simulink model "Simulador"  (R2015a)
settings: Solver=ode45  StartTime=0.0  StopTime=Inf  MaxStep=1  RelTol=1e-3
StopFcn:
  | close all
  | post_simulacion
model workspace (MAT data in the model file):
  m = 3.797
  b = 2.1
  c = 0.3571
  Salar = 0.75
  AR = 5.88
  cg = [0.44 0 0]
  Ix = 1.229
  Iy = 0.1702
  Iz = 0.8808
  Ixz = 0.9343
  e = 0.9935
  alpha0 = 0.267
  coefprop = [0.016415 -0.0142726]
  C_L0 = 0.0254
  C_Lalpha = 4.0191
  C_Lq = 3.8954
  C_Ldelta_e = 0.5872
  C_D0 = 0.0102
  C_Dbeta1 = -2.0864e-07
  C_Dbeta2 = 0.0671
  C_Dq = 0
  C_Ddelta_e = 0.8461
  C_Y0 = 3.2049e-18
  C_Ybeta = -0.1949
  C_Yp = -0.1172
  C_Yr = 0.0959
  C_Ydelta_a = -0.0696
  C_l0 = 1.1518e-18
  C_lbeta = -0.0765
  C_lp = -0.4018
  C_lr = 0.025
  C_ldelta_a = 0.2987
  C_m0 = 0.018
  C_malpha = -0.2524
  C_mq = -1.3047
  C_mdelta_e = -0.4857
  C_n0 = -2.2667e-07
  C_nbeta = 0.0403
  C_np = -0.0247
  C_nr = -0.1252
  C_ndelta_a = 0.0076
  gamma = 0.20958671
  gamma1 = 8.64638926772
  gamma2 = 7.15127867602
  gamma3 = 4.20255654569
  gamma4 = 4.4578208227
  gamma5 = -2.04582843713
  gamma6 = 5.48942420682
  gamma7 = 10.3736620037
  gamma8 = 5.86392142899
  C_p0 = -1.01045424588e-06
  C_pbeta = -0.14184539659
  C_pp = -1.79869539438
  C_pr = -0.45305525336
  C_pdelta_a = 1.28918307845
  C_r0 = -1.3291750703e-06
  C_rbeta = -0.104707259349
  C_rp = -1.93599126586
  C_rr = -0.622717442342
  C_rdelta_a = 1.3761168826
  C_mp = -0.2168
values from neighbouring files (symbols this model uses):
  r = [r_n;r_e;r_d]    [segmento.m]
  waypoints = reshape(waypoints_mat.',[],1)    [plan_de_vuelo.m]
undefined symbols (not defined in the file or in its folder): F, Light, magnitude, MIL, plan_de_vuelo
libraries: simulink_extras x20, aerolibconvert2 x18, aerolibfltsims x2, simulink x2, vrlib x1, instrumentlib x1, aerolibatmos2 x1, aerolibtransform2 x1, aerolibwind2 x1, aerolibgravity2 x1
(part 3 of 3)

== system Simulador/Autopiloto/Activador de controladores/Interruptor con latch/Memoria de pulsacion del teclado ==
  Estado del boton : Inport
  Reinicio : Inport  Port=2
  Activador : EnablePort
  Interruptor : Switch  Threshold=1
  Latch D : simulink_extras/Flip Flops/D Latch
  Memoria : Memory
  Operador logico : Logic  Operator=XOR  AllPortsSameDT=off  OutDataTypeStr=boolean
  Operador logico1 : Logic  AllPortsSameDT=off  OutDataTypeStr=boolean
  Operador logico2 : Logic  Operator=NOT  AllPortsSameDT=off  OutDataTypeStr=boolean
  Terminador : Terminator
  Tierra : Ground
  Estado del controlador : Outport
  wires:
  Operador logico2/1 -> Latch D/1
  Memoria/1 -> Operador logico2/1, Operador logico1/2
  Tierra/1 -> Interruptor/3
  Latch D/2 -> Terminador/1
  Estado del boton/1 -> Interruptor/2, Interruptor/1
  Latch D/1 -> Estado del controlador/1, Memoria/1
  Operador logico/1 -> Latch D/2
  Interruptor/1 -> Operador logico/1
  Reinicio/1 -> Operador logico1/1
  Operador logico1/1 -> Operador logico/2

== system Simulador/Autopiloto/Activador de controladores/Interruptor con latch1/Memoria de pulsacion del joystick ==
  Estado del boton : Inport
  Reinicio : Inport  Port=2
  Activador : EnablePort
  Interruptor1 : Switch  Criteria=u2 > Threshold
  Interruptor2 : Switch  Criteria=u2 > Threshold
  Latch D : simulink_extras/Flip Flops/D Latch
  Operador logico : Logic  Operator=NOT  AllPortsSameDT=off  OutDataTypeStr=boolean
  Operador logico1 : Logic  Operator=NOT  AllPortsSameDT=off  OutDataTypeStr=boolean
  Operador logico2 : Logic  Operator=XOR  AllPortsSameDT=off  OutDataTypeStr=boolean
  Retraso : Delay  DelayLength=1  InitialCondition=0  SampleTime=0.5
  Terminador : Terminator
  Estado del controlador : Outport
  wires:
  Latch D/2 -> Terminador/1
  Latch D/1 -> Retraso/1, Estado del controlador/1
  Operador logico/1 -> Interruptor1/1
  Retraso/1 -> Interruptor1/2
  Estado del boton/1 -> Operador logico/1, Interruptor1/3, Operador logico2/1
  Interruptor2/1 -> Latch D/1
  Interruptor1/1 -> Interruptor2/3
  Operador logico1/1 -> Interruptor2/1
  Operador logico2/1 -> Latch D/2
  Reinicio/1 -> Interruptor2/2, Operador logico1/1, Operador logico2/2

== system Simulador/Autopiloto/Activador de controladores/Interruptor con latch1/Memoria de pulsacion del teclado ==
  Estado del boton : Inport
  Reinicio : Inport  Port=2
  Activador : EnablePort
  Interruptor : Switch  Threshold=1
  Latch D : simulink_extras/Flip Flops/D Latch
  Memoria : Memory
  Operador logico : Logic  Operator=XOR  AllPortsSameDT=off  OutDataTypeStr=boolean
  Operador logico1 : Logic  AllPortsSameDT=off  OutDataTypeStr=boolean
  Operador logico2 : Logic  Operator=NOT  AllPortsSameDT=off  OutDataTypeStr=boolean
  Terminador : Terminator
  Tierra : Ground
  Estado del controlador : Outport
  wires:
  Operador logico2/1 -> Latch D/1
  Memoria/1 -> Operador logico2/1, Operador logico1/2
  Tierra/1 -> Interruptor/3
  Latch D/2 -> Terminador/1
  Estado del boton/1 -> Interruptor/2, Interruptor/1
  Latch D/1 -> Estado del controlador/1, Memoria/1
  Operador logico/1 -> Latch D/2
  Interruptor/1 -> Operador logico/1
  Reinicio/1 -> Operador logico1/1
  Operador logico1/1 -> Operador logico/2

== system Simulador/Autopiloto/Activador de controladores/Interruptor con latch2/Memoria de pulsacion del joystick ==
  Estado del boton : Inport
  Reinicio : Inport  Port=2
  Activador : EnablePort
  Interruptor1 : Switch  Criteria=u2 > Threshold
  Interruptor2 : Switch  Criteria=u2 > Threshold
  Latch D : simulink_extras/Flip Flops/D Latch
  Operador logico : Logic  Operator=NOT  AllPortsSameDT=off  OutDataTypeStr=boolean
  Operador logico1 : Logic  Operator=NOT  AllPortsSameDT=off  OutDataTypeStr=boolean
  Operador logico2 : Logic  Operator=XOR  AllPortsSameDT=off  OutDataTypeStr=boolean
  Retraso : Delay  DelayLength=1  InitialCondition=0  SampleTime=0.5
  Terminador : Terminator
  Estado del controlador : Outport
  wires:
  Latch D/2 -> Terminador/1
  Latch D/1 -> Retraso/1, Estado del controlador/1
  Operador logico/1 -> Interruptor1/1
  Retraso/1 -> Interruptor1/2
  Estado del boton/1 -> Operador logico/1, Interruptor1/3, Operador logico2/1
  Interruptor2/1 -> Latch D/1
  Interruptor1/1 -> Interruptor2/3
  Operador logico1/1 -> Interruptor2/1
  Operador logico2/1 -> Latch D/2
  Reinicio/1 -> Interruptor2/2, Operador logico1/1, Operador logico2/2

== system Simulador/Autopiloto/Activador de controladores/Interruptor con latch2/Memoria de pulsacion del teclado ==
  Estado del boton : Inport
  Reinicio : Inport  Port=2
  Activador : EnablePort
  Interruptor : Switch  Threshold=1
  Latch D : simulink_extras/Flip Flops/D Latch
  Memoria : Memory
  Operador logico : Logic  Operator=XOR  AllPortsSameDT=off  OutDataTypeStr=boolean
  Operador logico1 : Logic  AllPortsSameDT=off  OutDataTypeStr=boolean
  Operador logico2 : Logic  Operator=NOT  AllPortsSameDT=off  OutDataTypeStr=boolean
  Terminador : Terminator
  Tierra : Ground
  Estado del controlador : Outport
  wires:
  Operador logico2/1 -> Latch D/1
  Memoria/1 -> Operador logico2/1, Operador logico1/2
  Tierra/1 -> Interruptor/3
  Latch D/2 -> Terminador/1
  Estado del boton/1 -> Interruptor/2, Interruptor/1
  Latch D/1 -> Estado del controlador/1, Memoria/1
  Operador logico/1 -> Latch D/2
  Interruptor/1 -> Operador logico/1
  Reinicio/1 -> Operador logico1/1
  Operador logico1/1 -> Operador logico/2

== system Simulador/Autopiloto/Activador de controladores/Interruptor con latch3/Memoria de pulsacion del joystick ==
  Estado del boton : Inport
  Reinicio : Inport  Port=2
  Activador : EnablePort
  Interruptor1 : Switch  Criteria=u2 > Threshold
  Interruptor2 : Switch  Criteria=u2 > Threshold
  Latch D : simulink_extras/Flip Flops/D Latch
  Operador logico : Logic  Operator=NOT  AllPortsSameDT=off  OutDataTypeStr=boolean
  Operador logico1 : Logic  Operator=NOT  AllPortsSameDT=off  OutDataTypeStr=boolean
  Operador logico2 : Logic  Operator=XOR  AllPortsSameDT=off  OutDataTypeStr=boolean
  Retraso : Delay  DelayLength=1  InitialCondition=0  SampleTime=0.5
  Terminador : Terminator
  Estado del controlador : Outport
  wires:
  Latch D/2 -> Terminador/1
  Latch D/1 -> Retraso/1, Estado del controlador/1
  Operador logico/1 -> Interruptor1/1
  Retraso/1 -> Interruptor1/2
  Estado del boton/1 -> Operador logico/1, Interruptor1/3, Operador logico2/1
  Interruptor2/1 -> Latch D/1
  Interruptor1/1 -> Interruptor2/3
  Operador logico1/1 -> Interruptor2/1
  Operador logico2/1 -> Latch D/2
  Reinicio/1 -> Interruptor2/2, Operador logico1/1, Operador logico2/2

== system Simulador/Autopiloto/Activador de controladores/Interruptor con latch3/Memoria de pulsacion del teclado ==
  Estado del boton : Inport
  Reinicio : Inport  Port=2
  Activador : EnablePort
  Interruptor : Switch  Threshold=1
  Latch D : simulink_extras/Flip Flops/D Latch
  Memoria : Memory
  Operador logico : Logic  Operator=XOR  AllPortsSameDT=off  OutDataTypeStr=boolean
  Operador logico1 : Logic  AllPortsSameDT=off  OutDataTypeStr=boolean
  Operador logico2 : Logic  Operator=NOT  AllPortsSameDT=off  OutDataTypeStr=boolean
  Terminador : Terminator
  Tierra : Ground
  Estado del controlador : Outport
  wires:
  Operador logico2/1 -> Latch D/1
  Memoria/1 -> Operador logico2/1, Operador logico1/2
  Tierra/1 -> Interruptor/3
  Latch D/2 -> Terminador/1
  Estado del boton/1 -> Interruptor/2, Interruptor/1
  Latch D/1 -> Estado del controlador/1, Memoria/1
  Operador logico/1 -> Latch D/2
  Interruptor/1 -> Operador logico/1
  Reinicio/1 -> Operador logico1/1
  Operador logico1/1 -> Operador logico/2

== system Simulador/Autopiloto/Activador de controladores/Interruptor con latch4/Memoria de pulsacion del joystick ==
  Estado del boton : Inport
  Reinicio : Inport  Port=2
  Activador : EnablePort
  Interruptor1 : Switch  Criteria=u2 > Threshold
  Interruptor2 : Switch  Criteria=u2 > Threshold
  Latch D : simulink_extras/Flip Flops/D Latch
  Operador logico : Logic  Operator=NOT  AllPortsSameDT=off  OutDataTypeStr=boolean
  Operador logico1 : Logic  Operator=NOT  AllPortsSameDT=off  OutDataTypeStr=boolean
  Operador logico2 : Logic  Operator=XOR  AllPortsSameDT=off  OutDataTypeStr=boolean
  Retraso : Delay  DelayLength=1  InitialCondition=0  SampleTime=0.5
  Terminador : Terminator
  Estado del controlador : Outport
  wires:
  Latch D/2 -> Terminador/1
  Latch D/1 -> Retraso/1, Estado del controlador/1
  Operador logico/1 -> Interruptor1/1
  Retraso/1 -> Interruptor1/2
  Estado del boton/1 -> Operador logico/1, Interruptor1/3, Operador logico2/1
  Interruptor2/1 -> Latch D/1
  Interruptor1/1 -> Interruptor2/3
  Operador logico1/1 -> Interruptor2/1
  Operador logico2/1 -> Latch D/2
  Reinicio/1 -> Interruptor2/2, Operador logico1/1, Operador logico2/2

== system Simulador/Autopiloto/Activador de controladores/Interruptor con latch4/Memoria de pulsacion del teclado ==
  Estado del boton : Inport
  Reinicio : Inport  Port=2
  Activador : EnablePort
  Interruptor : Switch  Threshold=1
  Latch D : simulink_extras/Flip Flops/D Latch
  Memoria : Memory
  Operador logico : Logic  Operator=XOR  AllPortsSameDT=off  OutDataTypeStr=boolean
  Operador logico1 : Logic  AllPortsSameDT=off  OutDataTypeStr=boolean
  Operador logico2 : Logic  Operator=NOT  AllPortsSameDT=off  OutDataTypeStr=boolean
  Terminador : Terminator
  Tierra : Ground
  Estado del controlador : Outport
  wires:
  Operador logico2/1 -> Latch D/1
  Memoria/1 -> Operador logico2/1, Operador logico1/2
  Tierra/1 -> Interruptor/3
  Latch D/2 -> Terminador/1
  Estado del boton/1 -> Interruptor/2, Interruptor/1
  Latch D/1 -> Estado del controlador/1, Memoria/1
  Operador logico/1 -> Latch D/2
  Interruptor/1 -> Operador logico/1
  Reinicio/1 -> Operador logico1/1
  Operador logico1/1 -> Operador logico/2

== system Simulador/Autopiloto/Activador de controladores/Interruptor con latch5/Memoria de pulsacion del joystick ==
  Estado del boton : Inport
  Reinicio : Inport  Port=2
  Activador : EnablePort
  Interruptor1 : Switch  Criteria=u2 > Threshold
  Interruptor2 : Switch  Criteria=u2 > Threshold
  Latch D : simulink_extras/Flip Flops/D Latch
  Operador logico : Logic  Operator=NOT  AllPortsSameDT=off  OutDataTypeStr=boolean
  Operador logico1 : Logic  Operator=NOT  AllPortsSameDT=off  OutDataTypeStr=boolean
  Operador logico2 : Logic  Operator=XOR  AllPortsSameDT=off  OutDataTypeStr=boolean
  Retraso : Delay  DelayLength=1  InitialCondition=0  SampleTime=0.5
  Terminador : Terminator
  Estado del controlador : Outport
  wires:
  Latch D/2 -> Terminador/1
  Latch D/1 -> Retraso/1, Estado del controlador/1
  Operador logico/1 -> Interruptor1/1
  Retraso/1 -> Interruptor1/2
  Estado del boton/1 -> Operador logico/1, Interruptor1/3, Operador logico2/1
  Interruptor2/1 -> Latch D/1
  Interruptor1/1 -> Interruptor2/3
  Operador logico1/1 -> Interruptor2/1
  Operador logico2/1 -> Latch D/2
  Reinicio/1 -> Interruptor2/2, Operador logico1/1, Operador logico2/2

== system Simulador/Autopiloto/Activador de controladores/Interruptor con latch5/Memoria de pulsacion del teclado ==
  Estado del boton : Inport
  Reinicio : Inport  Port=2
  Activador : EnablePort
  Interruptor : Switch  Threshold=1
  Latch D : simulink_extras/Flip Flops/D Latch
  Memoria : Memory
  Operador logico : Logic  Operator=XOR  AllPortsSameDT=off  OutDataTypeStr=boolean
  Operador logico1 : Logic  AllPortsSameDT=off  OutDataTypeStr=boolean
  Operador logico2 : Logic  Operator=NOT  AllPortsSameDT=off  OutDataTypeStr=boolean
  Terminador : Terminator
  Tierra : Ground
  Estado del controlador : Outport
  wires:
  Operador logico2/1 -> Latch D/1
  Memoria/1 -> Operador logico2/1, Operador logico1/2
  Tierra/1 -> Interruptor/3
  Latch D/2 -> Terminador/1
  Estado del boton/1 -> Interruptor/2, Interruptor/1
  Latch D/1 -> Estado del controlador/1, Memoria/1
  Operador logico/1 -> Latch D/2
  Interruptor/1 -> Operador logico/1
  Reinicio/1 -> Operador logico1/1
  Operador logico1/1 -> Operador logico/2

== system Simulador/Autopiloto/Activador de controladores/Interruptor con latch6/Memoria de pulsacion del joystick ==
  Estado del boton : Inport
  Reinicio : Inport  Port=2
  Activador : EnablePort
  Interruptor1 : Switch  Criteria=u2 > Threshold
  Interruptor2 : Switch  Criteria=u2 > Threshold
  Latch D : simulink_extras/Flip Flops/D Latch
  Operador logico : Logic  Operator=NOT  AllPortsSameDT=off  OutDataTypeStr=boolean
  Operador logico1 : Logic  Operator=NOT  AllPortsSameDT=off  OutDataTypeStr=boolean
  Operador logico2 : Logic  Operator=XOR  AllPortsSameDT=off  OutDataTypeStr=boolean
  Retraso : Delay  DelayLength=1  InitialCondition=0  SampleTime=0.5
  Terminador : Terminator
  Estado del controlador : Outport
  wires:
  Latch D/2 -> Terminador/1
  Latch D/1 -> Retraso/1, Estado del controlador/1
  Operador logico/1 -> Interruptor1/1
  Retraso/1 -> Interruptor1/2
  Estado del boton/1 -> Operador logico/1, Interruptor1/3, Operador logico2/1
  Interruptor2/1 -> Latch D/1
  Interruptor1/1 -> Interruptor2/3
  Operador logico1/1 -> Interruptor2/1
  Operador logico2/1 -> Latch D/2
  Reinicio/1 -> Interruptor2/2, Operador logico1/1, Operador logico2/2

== system Simulador/Autopiloto/Activador de controladores/Interruptor con latch6/Memoria de pulsacion del teclado ==
  Estado del boton : Inport
  Reinicio : Inport  Port=2
  Activador : EnablePort
  Interruptor : Switch  Threshold=1
  Latch D : simulink_extras/Flip Flops/D Latch
  Memoria : Memory
  Operador logico : Logic  Operator=XOR  AllPortsSameDT=off  OutDataTypeStr=boolean
  Operador logico1 : Logic  AllPortsSameDT=off  OutDataTypeStr=boolean
  Operador logico2 : Logic  Operator=NOT  AllPortsSameDT=off  OutDataTypeStr=boolean
  Terminador : Terminator
  Tierra : Ground
  Estado del controlador : Outport
  wires:
  Operador logico2/1 -> Latch D/1
  Memoria/1 -> Operador logico2/1, Operador logico1/2
  Tierra/1 -> Interruptor/3
  Latch D/2 -> Terminador/1
  Estado del boton/1 -> Interruptor/2, Interruptor/1
  Latch D/1 -> Estado del controlador/1, Memoria/1
  Operador logico/1 -> Latch D/2
  Interruptor/1 -> Operador logico/1
  Reinicio/1 -> Operador logico1/1
  Operador logico1/1 -> Operador logico/2

== system Simulador/Autopiloto/Activador de controladores/Interruptor con latch7/Memoria de pulsacion del joystick ==
  Estado del boton : Inport
  Reinicio : Inport  Port=2
  Activador : EnablePort
  Interruptor1 : Switch  Criteria=u2 > Threshold
  Interruptor2 : Switch  Criteria=u2 > Threshold
  Latch D : simulink_extras/Flip Flops/D Latch
  Operador logico : Logic  Operator=NOT  AllPortsSameDT=off  OutDataTypeStr=boolean
  Operador logico1 : Logic  Operator=NOT  AllPortsSameDT=off  OutDataTypeStr=boolean
  Operador logico2 : Logic  Operator=XOR  AllPortsSameDT=off  OutDataTypeStr=boolean
  Retraso : Delay  DelayLength=1  InitialCondition=0  SampleTime=0.5
  Terminador : Terminator
  Estado del controlador : Outport
  wires:
  Latch D/2 -> Terminador/1
  Latch D/1 -> Retraso/1, Estado del controlador/1
  Operador logico/1 -> Interruptor1/1
  Retraso/1 -> Interruptor1/2
  Estado del boton/1 -> Operador logico/1, Interruptor1/3, Operador logico2/1
  Interruptor2/1 -> Latch D/1
  Interruptor1/1 -> Interruptor2/3
  Operador logico1/1 -> Interruptor2/1
  Operador logico2/1 -> Latch D/2
  Reinicio/1 -> Interruptor2/2, Operador logico1/1, Operador logico2/2

== system Simulador/Autopiloto/Activador de controladores/Interruptor con latch7/Memoria de pulsacion del teclado ==
  Estado del boton : Inport
  Reinicio : Inport  Port=2
  Activador : EnablePort
  Interruptor : Switch  Threshold=1
  Latch D : simulink_extras/Flip Flops/D Latch
  Memoria : Memory
  Operador logico : Logic  Operator=XOR  AllPortsSameDT=off  OutDataTypeStr=boolean
  Operador logico1 : Logic  AllPortsSameDT=off  OutDataTypeStr=boolean
  Operador logico2 : Logic  Operator=NOT  AllPortsSameDT=off  OutDataTypeStr=boolean
  Terminador : Terminator
  Tierra : Ground
  Estado del controlador : Outport
  wires:
  Operador logico2/1 -> Latch D/1
  Memoria/1 -> Operador logico2/1, Operador logico1/2
  Tierra/1 -> Interruptor/3
  Latch D/2 -> Terminador/1
  Estado del boton/1 -> Interruptor/2, Interruptor/1
  Latch D/1 -> Estado del controlador/1, Memoria/1
  Operador logico/1 -> Latch D/2
  Interruptor/1 -> Operador logico/1
  Reinicio/1 -> Operador logico1/1
  Operador logico1/1 -> Operador logico/2

== system Simulador/Autopiloto/Activador de controladores/Interruptor con latch8/Memoria de pulsacion del joystick ==
  Estado del boton : Inport
  Reinicio : Inport  Port=2
  Activador : EnablePort
  Interruptor1 : Switch  Criteria=u2 > Threshold
  Interruptor2 : Switch  Criteria=u2 > Threshold
  Latch D : simulink_extras/Flip Flops/D Latch
  Operador logico : Logic  Operator=NOT  AllPortsSameDT=off  OutDataTypeStr=boolean
  Operador logico1 : Logic  Operator=NOT  AllPortsSameDT=off  OutDataTypeStr=boolean
  Operador logico2 : Logic  Operator=XOR  AllPortsSameDT=off  OutDataTypeStr=boolean
  Retraso : Delay  DelayLength=1  InitialCondition=0  SampleTime=0.5
  Terminador : Terminator
  Estado del controlador : Outport
  wires:
  Latch D/2 -> Terminador/1
  Latch D/1 -> Retraso/1, Estado del controlador/1
  Operador logico/1 -> Interruptor1/1
  Retraso/1 -> Interruptor1/2
  Estado del boton/1 -> Operador logico/1, Interruptor1/3, Operador logico2/1
  Interruptor2/1 -> Latch D/1
  Interruptor1/1 -> Interruptor2/3
  Operador logico1/1 -> Interruptor2/1
  Operador logico2/1 -> Latch D/2
  Reinicio/1 -> Interruptor2/2, Operador logico1/1, Operador logico2/2

== system Simulador/Autopiloto/Activador de controladores/Interruptor con latch8/Memoria de pulsacion del teclado ==
  Estado del boton : Inport
  Reinicio : Inport  Port=2
  Activador : EnablePort
  Interruptor : Switch  Threshold=1
  Latch D : simulink_extras/Flip Flops/D Latch
  Memoria : Memory
  Operador logico : Logic  Operator=XOR  AllPortsSameDT=off  OutDataTypeStr=boolean
  Operador logico1 : Logic  AllPortsSameDT=off  OutDataTypeStr=boolean
  Operador logico2 : Logic  Operator=NOT  AllPortsSameDT=off  OutDataTypeStr=boolean
  Terminador : Terminator
  Tierra : Ground
  Estado del controlador : Outport
  wires:
  Operador logico2/1 -> Latch D/1
  Memoria/1 -> Operador logico2/1, Operador logico1/2
  Tierra/1 -> Interruptor/3
  Latch D/2 -> Terminador/1
  Estado del boton/1 -> Interruptor/2, Interruptor/1
  Latch D/1 -> Estado del controlador/1, Memoria/1
  Operador logico/1 -> Latch D/2
  Interruptor/1 -> Operador logico/1
  Reinicio/1 -> Operador logico1/1
  Operador logico1/1 -> Operador logico/2

== system Simulador/Autopiloto/Activador de controladores/Interruptor con latch9/Memoria de pulsacion del joystick ==
  Estado del boton : Inport
  Reinicio : Inport  Port=2
  Activador : EnablePort
  Interruptor1 : Switch  Criteria=u2 > Threshold
  Interruptor2 : Switch  Criteria=u2 > Threshold
  Latch D : simulink_extras/Flip Flops/D Latch
  Operador logico : Logic  Operator=NOT  AllPortsSameDT=off  OutDataTypeStr=boolean
  Operador logico1 : Logic  Operator=NOT  AllPortsSameDT=off  OutDataTypeStr=boolean
  Operador logico2 : Logic  Operator=XOR  AllPortsSameDT=off  OutDataTypeStr=boolean
  Retraso : Delay  DelayLength=1  InitialCondition=0  SampleTime=0.5
  Terminador : Terminator
  Estado del controlador : Outport
  wires:
  Latch D/2 -> Terminador/1
  Latch D/1 -> Retraso/1, Estado del controlador/1
  Operador logico/1 -> Interruptor1/1
  Retraso/1 -> Interruptor1/2
  Estado del boton/1 -> Operador logico/1, Interruptor1/3, Operador logico2/1
  Interruptor2/1 -> Latch D/1
  Interruptor1/1 -> Interruptor2/3
  Operador logico1/1 -> Interruptor2/1
  Operador logico2/1 -> Latch D/2
  Reinicio/1 -> Interruptor2/2, Operador logico1/1, Operador logico2/2

== system Simulador/Autopiloto/Activador de controladores/Interruptor con latch9/Memoria de pulsacion del teclado ==
  Estado del boton : Inport
  Reinicio : Inport  Port=2
  Activador : EnablePort
  Interruptor : Switch  Threshold=1
  Latch D : simulink_extras/Flip Flops/D Latch
  Memoria : Memory
  Operador logico : Logic  Operator=XOR  AllPortsSameDT=off  OutDataTypeStr=boolean
  Operador logico1 : Logic  AllPortsSameDT=off  OutDataTypeStr=boolean
  Operador logico2 : Logic  Operator=NOT  AllPortsSameDT=off  OutDataTypeStr=boolean
  Terminador : Terminator
  Tierra : Ground
  Estado del controlador : Outport
  wires:
  Operador logico2/1 -> Latch D/1
  Memoria/1 -> Operador logico2/1, Operador logico1/2
  Tierra/1 -> Interruptor/3
  Latch D/2 -> Terminador/1
  Estado del boton/1 -> Interruptor/2, Interruptor/1
  Latch D/1 -> Estado del controlador/1, Memoria/1
  Operador logico/1 -> Latch D/2
  Interruptor/1 -> Operador logico/1
  Reinicio/1 -> Operador logico1/1
  Operador logico1/1 -> Operador logico/2

== system Simulador/Entrada de control manual/Teclado/Reconocedor de teclado/Subsistema de accion del interruptor de eventos ==
  Eje alerones : Inport
  Tecla : Inport  Port=2
  Puerto de accion : ActionPort  ActionType=case
  Constante : Constant  Value=0.05
  Constante1 : Constant  Value=-0.05
  Interruptor : Switch  Criteria=u2 > Threshold  Threshold=97
  Saturacion : Saturate  UpperLimit=1  LowerLimit=-1
  Sum : Sum  Inputs=|++
  Eje alerones_ : Outport
  wires:
  Tecla/1 -> Interruptor/2
  Constante1/1 -> Interruptor/3
  Constante/1 -> Interruptor/1
  Eje alerones/1 -> Sum/1
  Interruptor/1 -> Sum/2
  Sum/1 -> Saturacion/1
  Saturacion/1 -> Eje alerones_/1

== system Simulador/Entrada de control manual/Teclado/Reconocedor de teclado/Subsistema de accion del interruptor de eventos1 ==
  Eje elevadores : Inport
  Tecla : Inport  Port=2
  Puerto de accion : ActionPort  ActionType=case
  Constante : Constant  Value=0.05
  Constante1 : Constant  Value=-0.05
  Interruptor : Switch  Criteria=u2 > Threshold  Threshold=115
  Saturacion : Saturate  UpperLimit=1  LowerLimit=-1
  Sum : Sum  Inputs=|++
  Eje elevadores_ : Outport
  wires:
  Eje elevadores/1 -> Sum/1
  Interruptor/1 -> Sum/2
  Sum/1 -> Saturacion/1
  Saturacion/1 -> Eje elevadores_/1
  Tecla/1 -> Interruptor/2
  Constante/1 -> Interruptor/1
  Constante1/1 -> Interruptor/3

== system Simulador/Entrada de control manual/Teclado/Reconocedor de teclado/Subsistema de accion del interruptor de eventos10 ==
  Pulsacion : Inport  PortDimensions=1
  Puerto de accion : ActionPort  ActionType=case
  Boton_ : Outport
  wires:
  Pulsacion/1 -> Boton_/1

== system Simulador/Entrada de control manual/Teclado/Reconocedor de teclado/Subsistema de accion del interruptor de eventos11 ==
  Pulsacion : Inport  PortDimensions=1
  Puerto de accion : ActionPort  ActionType=case
  Boton_ : Outport
  wires:
  Pulsacion/1 -> Boton_/1

== system Simulador/Entrada de control manual/Teclado/Reconocedor de teclado/Subsistema de accion del interruptor de eventos12 ==
  Pulsacion : Inport  PortDimensions=1
  Puerto de accion : ActionPort  ActionType=case
  Boton_ : Outport
  wires:
  Pulsacion/1 -> Boton_/1

== system Simulador/Entrada de control manual/Teclado/Reconocedor de teclado/Subsistema de accion del interruptor de eventos13 ==
  Pulsacion : Inport  PortDimensions=1
  Puerto de accion : ActionPort  ActionType=case
  Boton_ : Outport
  wires:
  Pulsacion/1 -> Boton_/1

== system Simulador/Entrada de control manual/Teclado/Reconocedor de teclado/Subsistema de accion del interruptor de eventos2 ==
  Eje motor : Inport
  Tecla : Inport  Port=2
  Puerto de accion : ActionPort  ActionType=case
  Constante : Constant  Value=-0.1
  Constante1 : Constant  Value=0.1
  Interruptor : Switch  Criteria=u2 > Threshold  Threshold=102
  Saturacion : Saturate  UpperLimit=1  LowerLimit=-1
  Sum : Sum  Inputs=|++
  Eje motor_ : Outport
  wires:
  Tecla/1 -> Interruptor/2
  Eje motor/1 -> Sum/1
  Interruptor/1 -> Sum/2
  Sum/1 -> Saturacion/1
  Saturacion/1 -> Eje motor_/1
  Constante1/1 -> Interruptor/3
  Constante/1 -> Interruptor/1

== system Simulador/Entrada de control manual/Teclado/Reconocedor de teclado/Subsistema de accion del interruptor de eventos3 ==
  Pulsacion : Inport  PortDimensions=1
  Puerto de accion : ActionPort  ActionType=case
  Boton_ : Outport
  wires:
  Pulsacion/1 -> Boton_/1

== system Simulador/Entrada de control manual/Teclado/Reconocedor de teclado/Subsistema de accion del interruptor de eventos4 ==
  Pulsacion : Inport  PortDimensions=1
  Puerto de accion : ActionPort  ActionType=case
  Boton_ : Outport
  wires:
  Pulsacion/1 -> Boton_/1

== system Simulador/Entrada de control manual/Teclado/Reconocedor de teclado/Subsistema de accion del interruptor de eventos5 ==
  Pulsacion : Inport  PortDimensions=1
  Puerto de accion : ActionPort  ActionType=case
  Boton_ : Outport
  wires:
  Pulsacion/1 -> Boton_/1

== system Simulador/Entrada de control manual/Teclado/Reconocedor de teclado/Subsistema de accion del interruptor de eventos6 ==
  Pulsacion : Inport  PortDimensions=1
  Puerto de accion : ActionPort  ActionType=case
  Boton_ : Outport
  wires:
  Pulsacion/1 -> Boton_/1

== system Simulador/Entrada de control manual/Teclado/Reconocedor de teclado/Subsistema de accion del interruptor de eventos7 ==
  Pulsacion : Inport  PortDimensions=1
  Puerto de accion : ActionPort  ActionType=case
  Boton_ : Outport
  wires:
  Pulsacion/1 -> Boton_/1

== system Simulador/Entrada de control manual/Teclado/Reconocedor de teclado/Subsistema de accion del interruptor de eventos8 ==
  Pulsacion : Inport  PortDimensions=1
  Puerto de accion : ActionPort  ActionType=case
  Boton_ : Outport
  wires:
  Pulsacion/1 -> Boton_/1

== system Simulador/Entrada de control manual/Teclado/Reconocedor de teclado/Subsistema de accion del interruptor de eventos9 ==
  Pulsacion : Inport  PortDimensions=1
  Puerto de accion : ActionPort  ActionType=case
  Boton_ : Outport
  wires:
  Pulsacion/1 -> Boton_/1
